simulink model "signal_gen_test"  (R2024a)
settings: Solver=VariableStepAuto  StartTime=0.0  StopTime=0.5  RelTol=1e-3
libraries: dsphdlxfrm2 x1
settings Model: Creator=Jan Rosa  LastModifiedBy=Jan Rosa

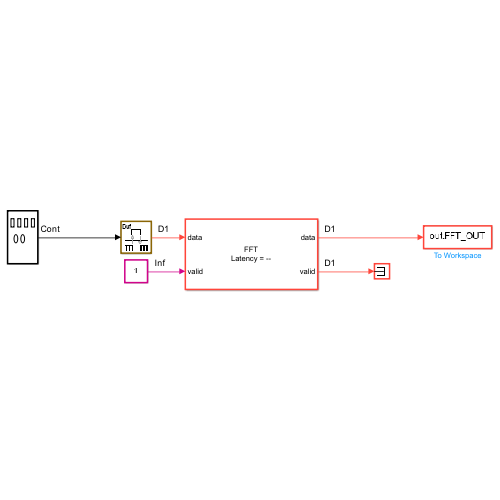
[thumbnail: Simulink's stored preview of the top-level diagram]
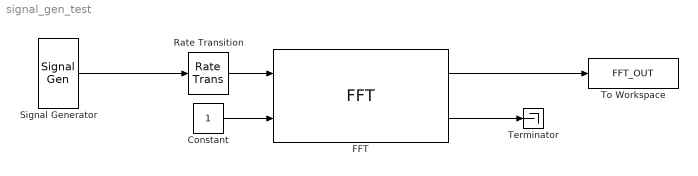
== system signal_gen_test ==
  Constant : Constant  OutDataTypeStr=boolean
  FFT : dsphdlxfrm2/FFT  Architecture=Streaming Radix 2^2  FFTLengthSource=Property  FFTLength=1024  FFTLengthMax=1024  ComplexMultiplication=Use 4 multipliers and 2 adders  BitReversedOutput=off  BitReversedInput=off  Normalize=off  SimulateUsing=Code generation  RoundingMethod=Floor  ResetInputPort=off  StartOutputPort=off  EndOutputPort=off
  Rate Transition : RateTransition  Deterministic=off  OutPortSampleTime=1/(50*16*16)
  Signal Generator : SignalGenerator  WaveForm=square  Frequency=50
  Terminator : Terminator
  To Workspace : ToWorkspace  VariableName=FFT_OUT  SaveFormat=Structure With Time  SampleTime=-1
  wires:
  Signal Generator/1 -> Rate Transition/1
  Rate Transition/1 -> FFT/1
  FFT/1 -> To Workspace/1
  Constant/1 -> FFT/2
  FFT/2 -> Terminator/1
